simulink model "Correction"  (R2021b)
settings: Solver=VariableStepAuto  StartTime=0.0  StopTime=10.0  RelTol=1e-3
settings Model: Creator=hugo  LastModifiedBy=hugo
settings SolverCC: AlgebraicLoopSolver=TrustRegion
settings DataIOCC: ReturnWorkspaceOutputs=off
settings DebuggingCC: SFMachineParentedDataDiag=warning  ArithmeticOperatorsInVariantConditions=warning
settings SFSimCC: SimUseLocalCustomCode=off  CustomCodeUndefinedFunction=UseInterfaceOnly
settings RTWCC: RTWUseLocalCustomCode=off

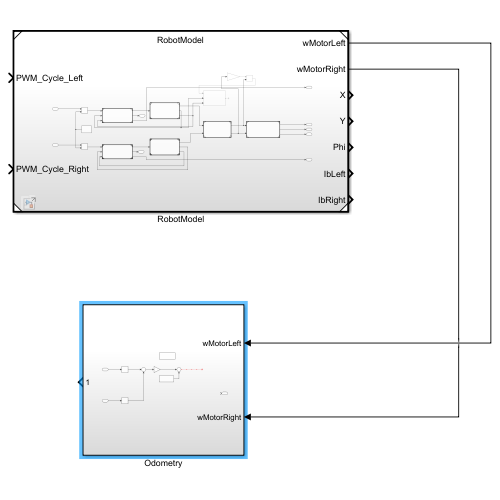
[thumbnail: Simulink's stored preview of the top-level diagram]
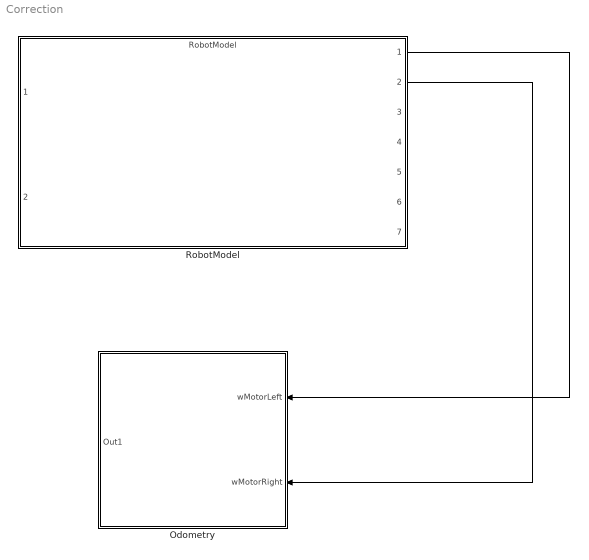
== system Correction ==
  Odometry : Subsystem
  RobotModel : ModelReference  ModelNameDialog=RobotModel.slx  SimulationMode=Normal  ModelReferenceVersion=1.60
  wires:
  RobotModel/1 -> Odometry/1(wMotorLeft)
  RobotModel/2 -> Odometry/2(wMotorRight)

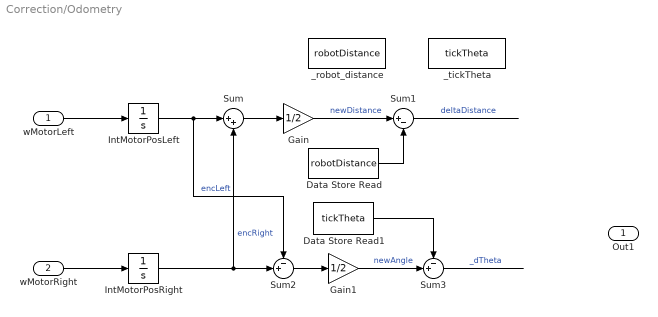
== system Correction/Odometry ==
  wMotorLeft : Inport
  wMotorRight : Inport  Port=2
  Data Store Read : DataStoreRead  DataStoreName=robotDistance  IndexOptions=Index vector (dialog)  Indices=1  OutputSizes=1
  Data Store Read1 : DataStoreRead  DataStoreName=tickTheta  IndexOptions=Index vector (dialog)  Indices=1  OutputSizes=1
  Gain : Gain  Gain=1/2
  Gain1 : Gain  Gain=1/2
  IntMotorPosLeft : Integrator  ContinuousStateAttributes='leftMotorAngle'
  IntMotorPosRight : Integrator  ContinuousStateAttributes='rightMotorAngle'
  Sum : Sum  Inputs=|++
  Sum1 : Sum  Inputs=|+-
  Sum2 : Sum  Inputs=-+|
  Sum3 : Sum  Inputs=-+|
  _robot_distance : DataStoreMemory  DataStoreName=robotDistance  ReadBeforeWriteMsg=warning  WriteAfterWriteMsg=warning  WriteAfterReadMsg=warning  ShowAdditionalParam=off
  _tickTheta : DataStoreMemory  DataStoreName=tickTheta  ReadBeforeWriteMsg=warning  WriteAfterWriteMsg=warning  WriteAfterReadMsg=warning  ShowAdditionalParam=off
  Out1 : Outport
  wires:
  wMotorLeft/1 -> IntMotorPosLeft/1
  wMotorRight/1 -> IntMotorPosRight/1
  IntMotorPosLeft/1 -> Sum2/1, Sum/1  "encLeft"
  IntMotorPosRight/1 -> Sum/2, Sum2/2  "encRight"
  Sum/1 -> Gain/1
  Gain/1 -> Sum1/1  "newDistance"
  Data Store Read/1 -> Sum1/2
  Sum1/1 -> ?  "deltaDistance"
  Sum2/1 -> Gain1/1
  Gain1/1 -> Sum3/2  "newAngle"
  Data Store Read1/1 -> Sum3/1
  Sum3/1 -> ?  "_dTheta"
